simulink model "dlbxzy"  (R2019b)
settings: Solver=FixedStepAuto  StartTime=0  StopTime=10.0  FixedStep=0.005  RelTol=1e-3  EnableMultiTasking=on
settings Model: Creator=guoyufan  LastModifiedBy=12603
settings DataIOCC: ReturnWorkspaceOutputs=off
settings OptimizationCC: LifeSpan=inf
settings DebuggingCC: SFUnexpectedBacktrackingDiag=warning  SFNoUnconditionalDefaultTransitionDiag=warning  ArithmeticOperatorsInVariantConditions=warning
settings SFSimCC: SimUseLocalCustomCode=off  CustomCodeUndefinedFunction=UseInterfaceOnly
settings RTWCC: RTWUseLocalCustomCode=off
settings CodeAppCC: StateflowObjectComments=on
settings GRTTargetCC: TargetLangStandard=C89/C90 (ANSI)  GeneratePreprocessorConditionals=Disable all
settings ConfigComp: CovMetricSettings=dw  CovHtmlReporting=on  CovSaveCumulativeToWorkspaceVar=on  CovSaveSingleToWorkspaceVar=on  CovExternalEMLEnable=off

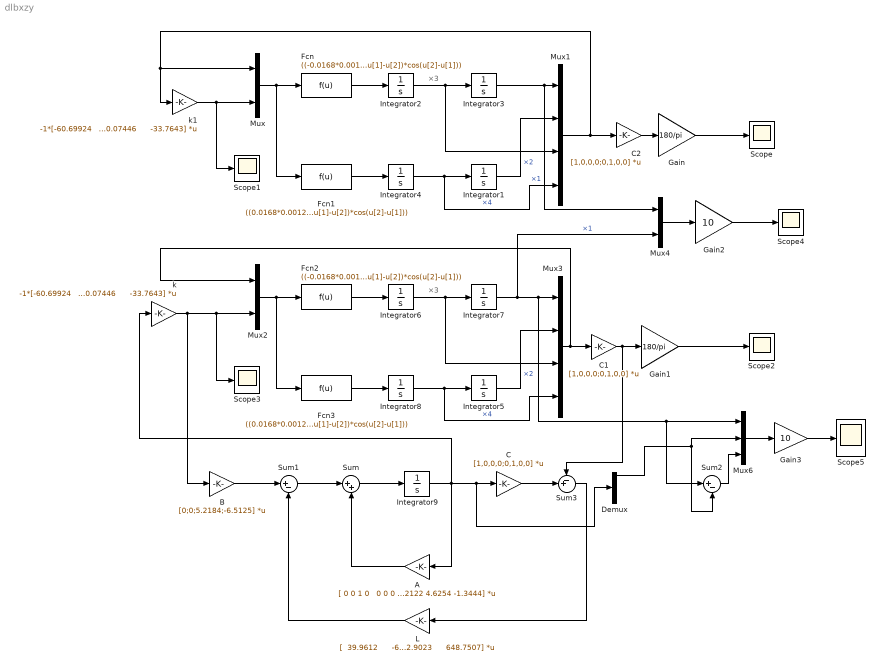
== system dlbxzy ==
  note: ×3
  note: ×3
  A : Gain  Gain=|  Multiplication=Matrix(K*u)
      | [ 0 0 1 0 
      |  0 0 0 1 
      |  65.8751 -16.8751 -3.7062 0.2760 
      |  -82.2122 82.2122 4.6254 -1.3444]
  B : Gain  Gain=[0;0;5.2184;-6.5125]  Multiplication=Matrix(K*u)
  C : Gain  Gain=[1,0,0,0;0,1,0,0]  Multiplication=Matrix(K*u)
  C1 : Gain  Gain=[1,0,0,0;0,1,0,0]  Multiplication=Matrix(K*u)
  C2 : Gain  Gain=[1,0,0,0;0,1,0,0]  Multiplication=Matrix(K*u)
  Demux : Demux
  Fcn : Fcn  Expr=((-0.0168*0.001)*u[3]+(0.001*0.0012*cos(u[2]-u[1]))*u[4]+0.0012*0.0012*sin(u[2]-u[1])* cos(u[2]-u[1])*u[3]*u[3]-0.0012*0.001*sin(u[1]-u[2])*u[4]*u[4]+0.2979*0.001*sin(u[1])-0.0612*0.0012*sin(u[2])*cos(u[2]-u[1])+0.0236*0.001*u[5])/(0.0061*0.001-0.0012*0.0012*cos(u[1]-u[2])*cos(u[2]-u[1]))
  Fcn1 : Fcn  Expr=((0.0168*0.0012*cos(u[1]-u[2]))*u[3]-(0.0061*0.001)*u[4]-0.0061*0.0012*sin(u[2]-u[1])*u[3]*u[3]+0.0012*0.0012*sin(u[1]-u[2])*cos(u[1]-u[2])*u[4]*u[4]-0.2979*0.0012*sin(u[1])*cos(u[1]-u[2])+0.0061*0.0612*sin(u[2])-0.0012*cos(u[1]-u[2])*0.0236*u[5])/(0.0061*0.001-0.0012*0.0012*cos(u[1]-u[2])*cos(u[2]-u[1]))
  Fcn2 : Fcn  Expr=((-0.0168*0.001)*u[3]+(0.001*0.0012*cos(u[2]-u[1]))*u[4]+0.0012*0.0012*sin(u[2]-u[1])* cos(u[2]-u[1])*u[3]*u[3]-0.0012*0.001*sin(u[1]-u[2])*u[4]*u[4]+0.2979*0.001*sin(u[1])-0.0612*0.0012*sin(u[2])*cos(u[2]-u[1])+0.0236*0.001*u[5])/(0.0061*0.001-0.0012*0.0012*cos(u[1]-u[2])*cos(u[2]-u[1]))
  Fcn3 : Fcn  Expr=((0.0168*0.0012*cos(u[1]-u[2]))*u[3]-(0.0061*0.001)*u[4]-0.0061*0.0012*sin(u[2]-u[1])*u[3]*u[3]+0.0012*0.0012*sin(u[1]-u[2])*cos(u[1]-u[2])*u[4]*u[4]-0.2979*0.0012*sin(u[1])*cos(u[1]-u[2])+0.0061*0.0612*sin(u[2])-0.0012*cos(u[1]-u[2])*0.0236*u[5])/(0.0061*0.001-0.0012*0.0012*cos(u[1]-u[2])*cos(u[2]-u[1]))
  Gain : Gain  Gain=180/pi
  Gain1 : Gain  Gain=180/pi
  Gain2 : Gain  Gain=10
  Gain3 : Gain  Gain=10
  Integrator1 : Integrator  InitialCondition=0.04
  Integrator{2,4,6,8..9} (5 alike) : Integrator
  Integrator3 : Integrator  InitialCondition=-0.06
  Integrator5 : Integrator  InitialCondition=0.04
  Integrator7 : Integrator  InitialCondition=-0.06
  L : Gain  Gain=|  Multiplication=Matrix(K*u)
      | [  39.9612      -60.4703
      | ; 0.697709       66.9882
      | ; 136.3525       443.818;
      | -152.9023      648.7507]
  Mux : Mux  Inputs=2
  Mux1 : Mux
  Mux2 : Mux  Inputs=2
  Mux3 : Mux
  Mux4 : Mux  Inputs=2
  Mux6 : Mux  Inputs=3
  Scope{,1..5} (6 alike) : Scope
  Sum : Sum  Inputs=|++
  Sum1 : Sum  Inputs=|+-
  Sum2 : Sum  Inputs=|+-
  Sum3 : Sum  Inputs=-+|
  k : Gain  Gain="-1*[-60.69924     -316.1745     -30.07446      -33.7643]"  Multiplication=Matrix(K*u)
  k1 : Gain  Gain="-1*[-60.69924     -316.1745     -30.07446      -33.7643]"  Multiplication=Matrix(K*u)
  wires:
  Mux/1 -> Fcn1/1, Fcn/1
  k1/1 -> Scope1/1, Mux/2
  Fcn/1 -> Integrator2/1
  Fcn1/1 -> Integrator4/1
  Integrator2/1 -> Mux1/3, Integrator3/1
  Integrator3/1 -> Mux4/1, Mux1/1  "×1"
  Integrator4/1 -> Mux1/4, Integrator1/1  "×4"
  Integrator1/1 -> Mux1/2  "×2"
  Gain/1 -> Scope/1
  Mux1/1 -> C2/1, Mux/1, k1/1
  Mux2/1 -> Fcn3/1, Fcn2/1
  k/1 -> B/1, Scope3/1, Mux2/2
  Fcn2/1 -> Integrator6/1
  Fcn3/1 -> Integrator8/1
  Integrator6/1 -> Mux3/3, Integrator7/1
  Integrator7/1 -> Mux4/2, Sum2/1, Mux6/1, Mux3/1  "×1"
  Integrator8/1 -> Mux3/4, Integrator5/1  "×4"
  Integrator5/1 -> Mux3/2  "×2"
  Gain1/1 -> Scope2/1
  Mux3/1 -> C1/1, Mux2/1
  C2/1 -> Gain/1
  C1/1 -> Gain1/1, Sum3/1
  Mux4/1 -> Gain2/1
  Gain2/1 -> Scope4/1
  B/1 -> Sum1/1
  Sum1/1 -> Sum/1
  Sum/1 -> Integrator9/1
  A/1 -> Sum/2
  L/1 -> Sum1/2
  C/1 -> Sum3/2
  Integrator9/1 -> Demux/1, C/1, k/1, A/1
  Sum3/1 -> L/1
  Sum2/1 -> Mux6/3
  Mux6/1 -> Gain3/1
  Gain3/1 -> Scope5/1
  Demux/1 -> Sum2/2, Mux6/2
